simulink model "HCS_Sim_r9_final"  (R2023a)
settings: Solver=ode4  StartTime=0.0  StopTime=24  FixedStep=5e-3  RelTol=1e-3  EnableMultiTasking=on
libraries: simulink x26, simulink_extras x11, arduinolib x8, spspowerguiLib x1
(part 2 of 5)

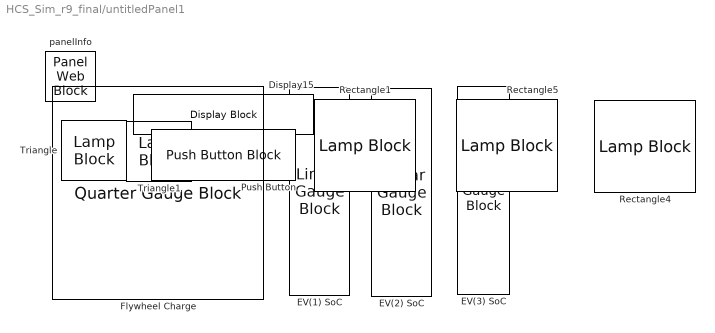
== system HCS_Sim_r9_final/untitledPanel1 ==
  Display15 : DisplayBlock  Tag=HiddenForWebPanel  PanelInfo="{\"height\":74,\"left\":296,\"panelId\":\"panelId-f3b1e18c-97eb-4ec7-afc3-1db5d88359af\",\"top\":88,\"type\":\"panelChild\",\"version\":\"2019b\",\"width\":182,\"zIndex\":1500022}"  LabelPosition=Hide  Format=bank  Alignment=Left  Transparency=1
  EV(1) SoC : LinearGaugeBlock  Tag=HiddenForWebPanel  PanelInfo="{\"height\":438,\"left\":576,\"panelId\":\"panelId-f3b1e18c-97eb-4ec7-afc3-1db5d88359af\",\"top\":279,\"type\":\"panelChild\",\"version\":\"2019b\",\"width\":116,\"zIndex\":1500004}"  LabelPosition=Hide  ScaleMax=1
  EV(2) SoC : LinearGaugeBlock  Tag=HiddenForWebPanel  PanelInfo="{\"height\":438,\"left\":830,\"panelId\":\"panelId-f3b1e18c-97eb-4ec7-afc3-1db5d88359af\",\"top\":279,\"type\":\"panelChild\",\"version\":\"2019b\",\"width\":128,\"zIndex\":1500006}"  LabelPosition=Hide  ScaleMax=1
  EV(3) SoC : LinearGaugeBlock  Tag=HiddenForWebPanel  PanelInfo="{\"height\":437,\"left\":1096,\"panelId\":\"panelId-f3b1e18c-97eb-4ec7-afc3-1db5d88359af\",\"top\":279,\"type\":\"panelChild\",\"version\":\"2019b\",\"width\":115,\"zIndex\":1500008}"  LabelPosition=Hide  ScaleMax=1
  Flywheel Charge : QuarterGaugeBlock  Tag=HiddenForWebPanel  PanelInfo="{\"height\":447,\"left\":56,\"panelId\":\"panelId-f3b1e18c-97eb-4ec7-afc3-1db5d88359af\",\"top\":268,\"type\":\"panelChild\",\"version\":\"2019b\",\"width\":444,\"zIndex\":1500010}"  LabelPosition=Hide  ScaleMax=45
  Push Button : PushButtonBlock  Tag=HiddenForWebPanel  PanelInfo="{\"height\":96,\"left\":227,\"panelId\":\"panelId-f3b1e18c-97eb-4ec7-afc3-1db5d88359af\",\"top\":175,\"type\":\"panelChild\",\"version\":\"2019b\",\"width\":270,\"zIndex\":1500024}"  ButtonText=Force Discharge  ButtonType=Latch  OffValue=0.000000
  Rectangle1 : LampBlock  Tag=HiddenForWebPanel  PanelInfo="{\"height\":172,\"left\":539,\"panelId\":\"panelId-f3b1e18c-97eb-4ec7-afc3-1db5d88359af\",\"top\":146,\"type\":\"panelChild\",\"version\":\"2019b\",\"width\":189,\"zIndex\":1500012}"  LabelPosition=Hide  Icon=Rectangle
  Rectangle4 : LampBlock  Tag=HiddenForWebPanel  PanelInfo="{\"height\":172,\"left\":1054,\"panelId\":\"panelId-f3b1e18c-97eb-4ec7-afc3-1db5d88359af\",\"top\":144,\"type\":\"panelChild\",\"version\":\"2019b\",\"width\":189,\"zIndex\":1500016}"  LabelPosition=Hide  Icon=Rectangle
  Rectangle5 : LampBlock  Tag=HiddenForWebPanel  PanelInfo="{\"height\":172,\"left\":794,\"panelId\":\"panelId-f3b1e18c-97eb-4ec7-afc3-1db5d88359af\",\"top\":144,\"type\":\"panelChild\",\"version\":\"2019b\",\"width\":189,\"zIndex\":1500014}"  LabelPosition=Hide  Icon=Rectangle
  Triangle : LampBlock  Tag=HiddenForWebPanel  PanelInfo="{\"height\":137,\"left\":27,\"panelId\":\"panelId-f3b1e18c-97eb-4ec7-afc3-1db5d88359af\",\"top\":163,\"type\":\"panelChild\",\"version\":\"2019b\",\"width\":151,\"zIndex\":1500018}"  LabelPosition=Hide  Icon=Triangle
  Triangle1 : LampBlock  Tag=HiddenForWebPanel  PanelInfo="{\"height\":137,\"left\":26,\"panelId\":\"panelId-f3b1e18c-97eb-4ec7-afc3-1db5d88359af\",\"top\":256,\"type\":\"panelChild\",\"version\":\"2019b\",\"width\":151,\"zIndex\":1500020}"  LabelPosition=Hide  Icon=Triangle
  panelInfo : PanelWebBlock  Tag=HiddenForWebPanel  PanelInfo="{\"compacted\":false,\"height\":800,\"isActiveTab\":false,\"labels\":{\"label2197221954\":{\"deleted\":false,\"left\":80,\"settings\":{\"backgroundColor\":\"rgba(0, 0, 0, 0)\",\"bold\":false,\"font\":\"Arial\",\"fontColor\":\"black\",\"fontSize\":1.68,\"italicized\":false,\"underlined\":false},\"text\":\"Simulation Time: \",\"top\":112},\"label4595339776\":{\"deleted\":false,\"left\":862,\"settings\":{\"backgroundColor\":\"rgba(0, 0, 0, 0)\",\"bold\":true,\"font\":\"Lucida Sans\",\"fontColor\":\"black\",\"fontSize\":1.48,\"italicized\":false,\"underlined\":false},\"text\":\"EV (2)\",\"top\":727},\"label4602337687\":{\"deleted\":false,\"left\":180,\"settings\":{\"backgroundColor\":\"rgba(0, 0, 0, 0)\",\"bold\":true,\"font\":\"Lucida Sans\",\"fontColor\":\"black\",\"fontSize\":1.68,\"italicized\":false,\"underlined\":false},\"text\":\"Flywheel (RPM)\",\"top\":727},\"label7574468105\":{\"deleted\":false,\"left\":601,\"settings\":{\"backgroundColor\":\"rgba(0, 0, 0, 0)\",\"bold\":true,\"font\":\"Lucida Sans\",\"fontColor\":\"black\",\"fontSize\":1.48,\"italicized\":false,\"underlined\":false},\"text\":\"EV (1)\",\"top\":727},\"label8183101307\":{\"deleted\":false,\"left\":1119,\"settings\":{\"backgroundColor\":\"rgba(0, 0, 0, 0)\",\"bold\":true,\"font\":\"Lucida Sans\",\"fontColor\":\"black\",\"fontSize\":1.48,\"italicized\":false,\"underlined\":false},\"text\":\"EV (3)\",\"top\":726},\"label8995571249\":{\"deleted\":false,\"left\":32,\"settings\":{\"backgroundColor\":\"rgba(0, 0, 0, 0)\",\"bold\":true,\"font\":\"Lucida Sans\",\"fontColor\":\"black\",\"fontSize\":2.62,\"italicized\":false,\"underlined\":false},\"text\":\"Flywheel & EV SoC Monitor\",\"top\":28}},\"left\":344,\"name\":\"Panel1\",\"panelId\":\"panelId-f3b1e18c-97eb-4ec7-afc3-1db5d88359af\",\"tabIndex\":1,\"tabbedSetId\":\"tabbedSet1419519353\",\"top\":42,\"type\":\"panel\",\"version\":\"2019b\",\"visible\":false,\"width\":1334,\"zIndex\":1500008}"  PanelSnapshot=<binary blob, 131972 chars, not shown>  PanelBackground=data:image/png;base64,iVBORw0KGgoAAAANSUhEUgAAAmYAAAHiCAYAAABC5QDZAAAAAXNSR0IArs4c6QAAAARnQU1BAACxjwv8YQUAAAAJcEhZcwAADsQAAA7EAZUrDhsAAAAZdEVYdFNvZnR3YXJlAEFkb2JlIEltYWdlUmVhZHlxyWU8AAADJGlUWHRYTUw6Y29tLmFkb2JlLnhtcAAAAAAAPD94cGFja2V0IGJlZ2luPSLvu78iIGlkPSJXNU0wTXBDZWhpSHpyZVN6TlRjemtjOWQiPz4gPHg6eG1wbWV0YSB4bWxuczp4PSJhZG9iZTpuczptZXRhLyIgeDp4bXB0az0iQWRvYmUgWE1QIENvcmUgNS4wLWMwNjEgNjQuMTQwOTQ5LCAyMDEwLzEyLzA3LTEwOjU3 ...(+5704 chars)
